simulink model "Proyecto_Final"  (R2025a)
settings: Solver=VariableStepAuto  StartTime=0.0  StopTime=10  RelTol=1e-3
undefined symbols (not defined in the file): X, Y, Z
libraries: fl_lib x336, nesl_utility x145, ee_lib x106, sm_lib x90, slpidlib x10
(part 2 of 13)

== system Proyecto_Final/Motor DC  ,Puente H y buck1 ==
  PS-Simulink Converter : nesl_utility/PS-Simulink Converter  PhysicalDomain=network_engine_domain  SubClassName=ps_output  LeftPortType=input  RightPortType=output  PseudoPeriodic=off  Frequencies=[]  VectorFormat=inherit  Unit=inherit  AffineConversion=off
  Scope3 : Scope
      settings: ActiveDisplayYMinimum=-1  ActiveDisplayYMaximum=1  DataLoggingVariableName=ScopeData11
  Subsystem : Subsystem
      settings: PortSchema="{\"entries\":[{\"content\":{\"sides\":[{\"content\":{\"connectorIds\":[\"LConn1\",\"LConn2\"]},\"type\":\"ConnectorPlacement.EquallySpacedRectSide\",\"uuid\":\"ba5a9f42-2585-4bfc-af33-0b26837d5344\"},{\"content\":{\"side\":\"RIGHT\"},\"type\":\"ConnectorPlacement.EquallySpacedRectSide\",\"uuid\":\"d3378d1a-9a35-4354-ae00-36e97aeae038\"},{\"content\":{\"connectorIds\":[\"LConn3\",\"LConn4\"],\"side\":\"TOP\"},\"type\":\"ConnectorPlacement.EquallySpacedRectSide\",\"uuid\":\"d7bba951-f995-49de-af79-0de620a32033\"}]},\"type\":\"ConnectorPlacement.EquallySpacedConnector\",\"uuid\":\"942587ed-ad52-4230-b73d-c158f6029d96\"}],\"packageUris\":[\"http://schema.mathworks.com/mf0/Connector/R2020b\"],\"version\":\"1.0\"}"
      mask Display: image('motordc.png');
  Subsystem1 : Subsystem
      mask Display: image('puenteh.png');
  Subsystem2 : Subsystem
      settings: PortSchema="{\"entries\":[{\"content\":{\"sides\":[{\"content\":{},\"type\":\"ConnectorPlacement.EquallySpacedRectSide\",\"uuid\":\"c0475787-e2dd-413a-bffe-1d488c503390\"},{\"content\":{\"connectorIds\":[\"RConn1\",\"RConn2\"],\"side\":\"RIGHT\"},\"type\":\"ConnectorPlacement.EquallySpacedRectSide\",\"uuid\":\"7136259c-9599-4eb8-8e1f-6288fad3fd4d\"},{\"content\":{\"side\":\"TOP\"},\"type\":\"ConnectorPlacement.EquallySpacedRectSide\",\"uuid\":\"c12a757b-7dec-4835-b4c8-0dd09d9bf8df\"},{\"content\":{\"connectorIds\":[\"RConn3\"],\"side\":\"BOTTOM\"},\"type\":\"ConnectorPlacement.EquallySpacedRectSide\",\"uuid\":\"8c834916-1092-4edf-bbd6-cfa333fcf008\"}]},\"type\":\"ConnectorPlacement.EquallySpacedConnector\",\"uuid\":\"4818e542-4a83-49f7-b80e-d9385aa09b38\"}],\"packageUris\":[\"http://schema.mathworks.com/mf0/Connector/R2020b\"],\"version\":\"1.0\"}"
      mask Display: image('buck.jpg');
  Voltage Sensor1 : fl_lib/Electrical/Electrical Sensors/Voltage Sensor
  w : PMIOPort  Side=Right
  t : PMIOPort  Port=2  Side=Right
  Lazo : PMIOPort  Port=3  Side=Right
  wires:
  PS-Simulink Converter/1 -> Scope3/1
  connections:
  Subsystem1/LConn1 -- Voltage Sensor1/LConn1 -- Subsystem2/RConn1
  Voltage Sensor1/RConn2 -- Subsystem1/LConn2 -- Subsystem2/RConn2
  Voltage Sensor1/RConn1 -- PS-Simulink Converter/LConn1
  w/RConn1 -- Subsystem/LConn4
  Subsystem/LConn3 -- t/RConn1
  Subsystem1/RConn1 -- Subsystem/LConn1
  Subsystem1/RConn2 -- Subsystem/LConn2
  Lazo/RConn1 -- Subsystem2/RConn3

== system Proyecto_Final/Motor DC  ,Puente H y buck2 ==
  PS-Simulink Converter : nesl_utility/PS-Simulink Converter  PhysicalDomain=network_engine_domain  SubClassName=ps_output  LeftPortType=input  RightPortType=output  PseudoPeriodic=off  Frequencies=[]  VectorFormat=inherit  Unit=inherit  AffineConversion=off
  Scope3 : Scope
      settings: ActiveDisplayYMinimum=-166.62843332082716  ActiveDisplayYMaximum=1034.7868051822825  DataLoggingVariableName=ScopeData33
  Subsystem : Subsystem
      settings: PortSchema="{\"entries\":[{\"content\":{\"sides\":[{\"content\":{\"connectorIds\":[\"LConn1\",\"LConn2\"]},\"type\":\"ConnectorPlacement.EquallySpacedRectSide\",\"uuid\":\"ba5a9f42-2585-4bfc-af33-0b26837d5344\"},{\"content\":{\"side\":\"RIGHT\"},\"type\":\"ConnectorPlacement.EquallySpacedRectSide\",\"uuid\":\"d3378d1a-9a35-4354-ae00-36e97aeae038\"},{\"content\":{\"connectorIds\":[\"LConn3\",\"LConn4\"],\"side\":\"TOP\"},\"type\":\"ConnectorPlacement.EquallySpacedRectSide\",\"uuid\":\"d7bba951-f995-49de-af79-0de620a32033\"}]},\"type\":\"ConnectorPlacement.EquallySpacedConnector\",\"uuid\":\"942587ed-ad52-4230-b73d-c158f6029d96\"}],\"packageUris\":[\"http://schema.mathworks.com/mf0/Connector/R2020b\"],\"version\":\"1.0\"}"
      mask Display: image('motordc.png');
  Subsystem1 : Subsystem
      mask Display: image('puenteh.png');
  Subsystem2 : Subsystem
      settings: PortSchema="{\"entries\":[{\"content\":{\"sides\":[{\"content\":{},\"type\":\"ConnectorPlacement.EquallySpacedRectSide\",\"uuid\":\"c0475787-e2dd-413a-bffe-1d488c503390\"},{\"content\":{\"connectorIds\":[\"RConn1\",\"RConn2\"],\"side\":\"RIGHT\"},\"type\":\"ConnectorPlacement.EquallySpacedRectSide\",\"uuid\":\"7136259c-9599-4eb8-8e1f-6288fad3fd4d\"},{\"content\":{\"side\":\"TOP\"},\"type\":\"ConnectorPlacement.EquallySpacedRectSide\",\"uuid\":\"c12a757b-7dec-4835-b4c8-0dd09d9bf8df\"},{\"content\":{\"connectorIds\":[\"RConn3\"],\"side\":\"BOTTOM\"},\"type\":\"ConnectorPlacement.EquallySpacedRectSide\",\"uuid\":\"8c834916-1092-4edf-bbd6-cfa333fcf008\"}]},\"type\":\"ConnectorPlacement.EquallySpacedConnector\",\"uuid\":\"4818e542-4a83-49f7-b80e-d9385aa09b38\"}],\"packageUris\":[\"http://schema.mathworks.com/mf0/Connector/R2020b\"],\"version\":\"1.0\"}"
      mask Display: image('buck.jpg');
  Voltage Sensor1 : fl_lib/Electrical/Electrical Sensors/Voltage Sensor
  w : PMIOPort  Side=Right
  t : PMIOPort  Port=2  Side=Right
  Lazo : PMIOPort  Port=3  Side=Right
  wires:
  PS-Simulink Converter/1 -> Scope3/1
  connections:
  Subsystem1/LConn2 -- Subsystem2/RConn2 -- Voltage Sensor1/RConn2
  Subsystem1/LConn1 -- Voltage Sensor1/LConn1 -- Subsystem2/RConn1
  Lazo/RConn1 -- Subsystem2/RConn3
  Subsystem1/RConn2 -- Subsystem/LConn2
  Subsystem/LConn3 -- t/RConn1
  Voltage Sensor1/RConn1 -- PS-Simulink Converter/LConn1
  w/RConn1 -- Subsystem/LConn4
  Subsystem1/RConn1 -- Subsystem/LConn1

== system Proyecto_Final/Motor DC  ,Puente H y buck3 ==
  PS-Simulink Converter : nesl_utility/PS-Simulink Converter  PhysicalDomain=network_engine_domain  SubClassName=ps_output  LeftPortType=input  RightPortType=output  PseudoPeriodic=off  Frequencies=[]  VectorFormat=inherit  Unit=inherit  AffineConversion=off
  Scope3 : Scope
      settings: ActiveDisplayYMinimum=-1  ActiveDisplayYMaximum=1  DataLoggingVariableName=ScopeData11
  Subsystem : Subsystem
      settings: PortSchema="{\"entries\":[{\"content\":{\"sides\":[{\"content\":{\"connectorIds\":[\"LConn1\",\"LConn2\"]},\"type\":\"ConnectorPlacement.EquallySpacedRectSide\",\"uuid\":\"ba5a9f42-2585-4bfc-af33-0b26837d5344\"},{\"content\":{\"side\":\"RIGHT\"},\"type\":\"ConnectorPlacement.EquallySpacedRectSide\",\"uuid\":\"d3378d1a-9a35-4354-ae00-36e97aeae038\"},{\"content\":{\"connectorIds\":[\"LConn3\",\"LConn4\"],\"side\":\"TOP\"},\"type\":\"ConnectorPlacement.EquallySpacedRectSide\",\"uuid\":\"d7bba951-f995-49de-af79-0de620a32033\"}]},\"type\":\"ConnectorPlacement.EquallySpacedConnector\",\"uuid\":\"942587ed-ad52-4230-b73d-c158f6029d96\"}],\"packageUris\":[\"http://schema.mathworks.com/mf0/Connector/R2020b\"],\"version\":\"1.0\"}"
      mask Display: image('motordc.png');
  Subsystem1 : Subsystem
      mask Display: image('puenteh.png');
  Subsystem2 : Subsystem
      settings: PortSchema="{\"entries\":[{\"content\":{\"sides\":[{\"content\":{},\"type\":\"ConnectorPlacement.EquallySpacedRectSide\",\"uuid\":\"c0475787-e2dd-413a-bffe-1d488c503390\"},{\"content\":{\"connectorIds\":[\"RConn1\",\"RConn2\"],\"side\":\"RIGHT\"},\"type\":\"ConnectorPlacement.EquallySpacedRectSide\",\"uuid\":\"7136259c-9599-4eb8-8e1f-6288fad3fd4d\"},{\"content\":{\"side\":\"TOP\"},\"type\":\"ConnectorPlacement.EquallySpacedRectSide\",\"uuid\":\"c12a757b-7dec-4835-b4c8-0dd09d9bf8df\"},{\"content\":{\"connectorIds\":[\"RConn3\"],\"side\":\"BOTTOM\"},\"type\":\"ConnectorPlacement.EquallySpacedRectSide\",\"uuid\":\"8c834916-1092-4edf-bbd6-cfa333fcf008\"}]},\"type\":\"ConnectorPlacement.EquallySpacedConnector\",\"uuid\":\"4818e542-4a83-49f7-b80e-d9385aa09b38\"}],\"packageUris\":[\"http://schema.mathworks.com/mf0/Connector/R2020b\"],\"version\":\"1.0\"}"
      mask Display: image('buck.jpg');
  Voltage Sensor1 : fl_lib/Electrical/Electrical Sensors/Voltage Sensor
  w : PMIOPort  Side=Right
  t : PMIOPort  Port=2  Side=Right
  Lazo : PMIOPort  Port=3  Side=Right
  wires:
  PS-Simulink Converter/1 -> Scope3/1
  connections:
  Voltage Sensor1/LConn1 -- Subsystem2/RConn1 -- Subsystem1/LConn1
  Voltage Sensor1/RConn2 -- Subsystem1/LConn2 -- Subsystem2/RConn2
  Voltage Sensor1/RConn1 -- PS-Simulink Converter/LConn1
  w/RConn1 -- Subsystem/LConn4
  Subsystem/LConn3 -- t/RConn1
  Subsystem1/RConn1 -- Subsystem/LConn1
  Subsystem1/RConn2 -- Subsystem/LConn2
  Lazo/RConn1 -- Subsystem2/RConn3

== system Proyecto_Final/Motor DC  ,Puente H y buck4 ==
  PS-Simulink Converter : nesl_utility/PS-Simulink Converter  PhysicalDomain=network_engine_domain  SubClassName=ps_output  LeftPortType=input  RightPortType=output  PseudoPeriodic=off  Frequencies=[]  VectorFormat=inherit  Unit=inherit  AffineConversion=off
  Scope3 : Scope
      settings: ActiveDisplayYMinimum=-166.62843332082716  ActiveDisplayYMaximum=1034.7868051822825  DataLoggingVariableName=ScopeData33
  Subsystem : Subsystem
      settings: PortSchema="{\"entries\":[{\"content\":{\"sides\":[{\"content\":{\"connectorIds\":[\"LConn1\",\"LConn2\"]},\"type\":\"ConnectorPlacement.EquallySpacedRectSide\",\"uuid\":\"ba5a9f42-2585-4bfc-af33-0b26837d5344\"},{\"content\":{\"side\":\"RIGHT\"},\"type\":\"ConnectorPlacement.EquallySpacedRectSide\",\"uuid\":\"d3378d1a-9a35-4354-ae00-36e97aeae038\"},{\"content\":{\"connectorIds\":[\"LConn3\",\"LConn4\"],\"side\":\"TOP\"},\"type\":\"ConnectorPlacement.EquallySpacedRectSide\",\"uuid\":\"d7bba951-f995-49de-af79-0de620a32033\"}]},\"type\":\"ConnectorPlacement.EquallySpacedConnector\",\"uuid\":\"942587ed-ad52-4230-b73d-c158f6029d96\"}],\"packageUris\":[\"http://schema.mathworks.com/mf0/Connector/R2020b\"],\"version\":\"1.0\"}"
      mask Display: image('motordc.png');
  Subsystem1 : Subsystem
      mask Display: image('puenteh.png');
  Subsystem2 : Subsystem
      settings: PortSchema="{\"entries\":[{\"content\":{\"sides\":[{\"content\":{},\"type\":\"ConnectorPlacement.EquallySpacedRectSide\",\"uuid\":\"c0475787-e2dd-413a-bffe-1d488c503390\"},{\"content\":{\"connectorIds\":[\"RConn1\",\"RConn2\"],\"side\":\"RIGHT\"},\"type\":\"ConnectorPlacement.EquallySpacedRectSide\",\"uuid\":\"7136259c-9599-4eb8-8e1f-6288fad3fd4d\"},{\"content\":{\"side\":\"TOP\"},\"type\":\"ConnectorPlacement.EquallySpacedRectSide\",\"uuid\":\"c12a757b-7dec-4835-b4c8-0dd09d9bf8df\"},{\"content\":{\"connectorIds\":[\"RConn3\"],\"side\":\"BOTTOM\"},\"type\":\"ConnectorPlacement.EquallySpacedRectSide\",\"uuid\":\"8c834916-1092-4edf-bbd6-cfa333fcf008\"}]},\"type\":\"ConnectorPlacement.EquallySpacedConnector\",\"uuid\":\"4818e542-4a83-49f7-b80e-d9385aa09b38\"}],\"packageUris\":[\"http://schema.mathworks.com/mf0/Connector/R2020b\"],\"version\":\"1.0\"}"
      mask Display: image('buck.jpg');
  Voltage Sensor1 : fl_lib/Electrical/Electrical Sensors/Voltage Sensor
  w : PMIOPort  Side=Right
  t : PMIOPort  Port=2  Side=Right
  Lazo : PMIOPort  Port=3  Side=Right
  wires:
  PS-Simulink Converter/1 -> Scope3/1
  connections:
  Subsystem2/RConn2 -- Voltage Sensor1/RConn2 -- Subsystem1/LConn2
  Voltage Sensor1/LConn1 -- Subsystem2/RConn1 -- Subsystem1/LConn1
  Lazo/RConn1 -- Subsystem2/RConn3
  Subsystem1/RConn2 -- Subsystem/LConn2
  Subsystem/LConn3 -- t/RConn1
  Voltage Sensor1/RConn1 -- PS-Simulink Converter/LConn1
  w/RConn1 -- Subsystem/LConn4
  Subsystem1/RConn1 -- Subsystem/LConn1

== system Proyecto_Final/Motor DC  ,Puente H y buck5 ==
  PS-Simulink Converter : nesl_utility/PS-Simulink Converter  PhysicalDomain=network_engine_domain  SubClassName=ps_output  LeftPortType=input  RightPortType=output  PseudoPeriodic=off  Frequencies=[]  VectorFormat=inherit  Unit=inherit  AffineConversion=off
  Scope3 : Scope
      settings: ActiveDisplayYMinimum=-166.62843332082716  ActiveDisplayYMaximum=1034.7868051822825  DataLoggingVariableName=ScopeData34
  Subsystem : Subsystem
      settings: PortSchema="{\"entries\":[{\"content\":{\"sides\":[{\"content\":{\"connectorIds\":[\"LConn1\",\"LConn2\"]},\"type\":\"ConnectorPlacement.EquallySpacedRectSide\",\"uuid\":\"ba5a9f42-2585-4bfc-af33-0b26837d5344\"},{\"content\":{\"side\":\"RIGHT\"},\"type\":\"ConnectorPlacement.EquallySpacedRectSide\",\"uuid\":\"d3378d1a-9a35-4354-ae00-36e97aeae038\"},{\"content\":{\"connectorIds\":[\"LConn3\",\"LConn4\"],\"side\":\"TOP\"},\"type\":\"ConnectorPlacement.EquallySpacedRectSide\",\"uuid\":\"d7bba951-f995-49de-af79-0de620a32033\"}]},\"type\":\"ConnectorPlacement.EquallySpacedConnector\",\"uuid\":\"942587ed-ad52-4230-b73d-c158f6029d96\"}],\"packageUris\":[\"http://schema.mathworks.com/mf0/Connector/R2020b\"],\"version\":\"1.0\"}"
      mask Display: image('motordc.png');
  Subsystem1 : Subsystem
      mask Display: image('puenteh.png');
  Subsystem2 : Subsystem
      settings: PortSchema="{\"entries\":[{\"content\":{\"sides\":[{\"content\":{},\"type\":\"ConnectorPlacement.EquallySpacedRectSide\",\"uuid\":\"c0475787-e2dd-413a-bffe-1d488c503390\"},{\"content\":{\"connectorIds\":[\"RConn1\",\"RConn2\"],\"side\":\"RIGHT\"},\"type\":\"ConnectorPlacement.EquallySpacedRectSide\",\"uuid\":\"7136259c-9599-4eb8-8e1f-6288fad3fd4d\"},{\"content\":{\"side\":\"TOP\"},\"type\":\"ConnectorPlacement.EquallySpacedRectSide\",\"uuid\":\"c12a757b-7dec-4835-b4c8-0dd09d9bf8df\"},{\"content\":{\"connectorIds\":[\"RConn3\"],\"side\":\"BOTTOM\"},\"type\":\"ConnectorPlacement.EquallySpacedRectSide\",\"uuid\":\"8c834916-1092-4edf-bbd6-cfa333fcf008\"}]},\"type\":\"ConnectorPlacement.EquallySpacedConnector\",\"uuid\":\"4818e542-4a83-49f7-b80e-d9385aa09b38\"}],\"packageUris\":[\"http://schema.mathworks.com/mf0/Connector/R2020b\"],\"version\":\"1.0\"}"
      mask Display: image('buck.jpg');
  Voltage Sensor1 : fl_lib/Electrical/Electrical Sensors/Voltage Sensor
  w : PMIOPort  Side=Right
  t : PMIOPort  Port=2  Side=Right
  Lazo : PMIOPort  Port=3  Side=Right
  wires:
  PS-Simulink Converter/1 -> Scope3/1
  connections:
  Subsystem2/RConn2 -- Voltage Sensor1/RConn2 -- Subsystem1/LConn2
  Voltage Sensor1/LConn1 -- Subsystem2/RConn1 -- Subsystem1/LConn1
  Lazo/RConn1 -- Subsystem2/RConn3
  Subsystem1/RConn2 -- Subsystem/LConn2
  Subsystem/LConn3 -- t/RConn1
  Voltage Sensor1/RConn1 -- PS-Simulink Converter/LConn1
  w/RConn1 -- Subsystem/LConn4
  Subsystem1/RConn1 -- Subsystem/LConn1

== system Proyecto_Final/Motor DC  ,Puente H y buck6 ==
  PS-Simulink Converter : nesl_utility/PS-Simulink Converter  PhysicalDomain=network_engine_domain  SubClassName=ps_output  LeftPortType=input  RightPortType=output  PseudoPeriodic=off  Frequencies=[]  VectorFormat=inherit  Unit=inherit  AffineConversion=off
  Scope3 : Scope
      settings: ActiveDisplayYMinimum=-166.62843332082716  ActiveDisplayYMaximum=1034.7868051822825  DataLoggingVariableName=ScopeData34
  Subsystem : Subsystem
      settings: PortSchema="{\"entries\":[{\"content\":{\"sides\":[{\"content\":{\"connectorIds\":[\"LConn1\",\"LConn2\"]},\"type\":\"ConnectorPlacement.EquallySpacedRectSide\",\"uuid\":\"ba5a9f42-2585-4bfc-af33-0b26837d5344\"},{\"content\":{\"side\":\"RIGHT\"},\"type\":\"ConnectorPlacement.EquallySpacedRectSide\",\"uuid\":\"d3378d1a-9a35-4354-ae00-36e97aeae038\"},{\"content\":{\"connectorIds\":[\"LConn3\",\"LConn4\"],\"side\":\"TOP\"},\"type\":\"ConnectorPlacement.EquallySpacedRectSide\",\"uuid\":\"d7bba951-f995-49de-af79-0de620a32033\"}]},\"type\":\"ConnectorPlacement.EquallySpacedConnector\",\"uuid\":\"942587ed-ad52-4230-b73d-c158f6029d96\"}],\"packageUris\":[\"http://schema.mathworks.com/mf0/Connector/R2020b\"],\"version\":\"1.0\"}"
      mask Display: image('motordc.png');
  Subsystem1 : Subsystem
      mask Display: image('puenteh.png');
  Subsystem2 : Subsystem
      settings: PortSchema="{\"entries\":[{\"content\":{\"sides\":[{\"content\":{},\"type\":\"ConnectorPlacement.EquallySpacedRectSide\",\"uuid\":\"c0475787-e2dd-413a-bffe-1d488c503390\"},{\"content\":{\"connectorIds\":[\"RConn1\",\"RConn2\"],\"side\":\"RIGHT\"},\"type\":\"ConnectorPlacement.EquallySpacedRectSide\",\"uuid\":\"7136259c-9599-4eb8-8e1f-6288fad3fd4d\"},{\"content\":{\"side\":\"TOP\"},\"type\":\"ConnectorPlacement.EquallySpacedRectSide\",\"uuid\":\"c12a757b-7dec-4835-b4c8-0dd09d9bf8df\"},{\"content\":{\"connectorIds\":[\"RConn3\"],\"side\":\"BOTTOM\"},\"type\":\"ConnectorPlacement.EquallySpacedRectSide\",\"uuid\":\"8c834916-1092-4edf-bbd6-cfa333fcf008\"}]},\"type\":\"ConnectorPlacement.EquallySpacedConnector\",\"uuid\":\"4818e542-4a83-49f7-b80e-d9385aa09b38\"}],\"packageUris\":[\"http://schema.mathworks.com/mf0/Connector/R2020b\"],\"version\":\"1.0\"}"
      mask Display: image('buck.jpg');
  Voltage Sensor1 : fl_lib/Electrical/Electrical Sensors/Voltage Sensor
  w : PMIOPort  Side=Right
  t : PMIOPort  Port=2  Side=Right
  Lazo : PMIOPort  Port=3  Side=Right
  wires:
  PS-Simulink Converter/1 -> Scope3/1
  connections:
  Subsystem1/LConn2 -- Subsystem2/RConn2 -- Voltage Sensor1/RConn2
  Subsystem1/LConn1 -- Voltage Sensor1/LConn1 -- Subsystem2/RConn1
  Lazo/RConn1 -- Subsystem2/RConn3
  Subsystem1/RConn2 -- Subsystem/LConn2
  Subsystem/LConn3 -- t/RConn1
  Voltage Sensor1/RConn1 -- PS-Simulink Converter/LConn1
  w/RConn1 -- Subsystem/LConn4
  Subsystem1/RConn1 -- Subsystem/LConn1

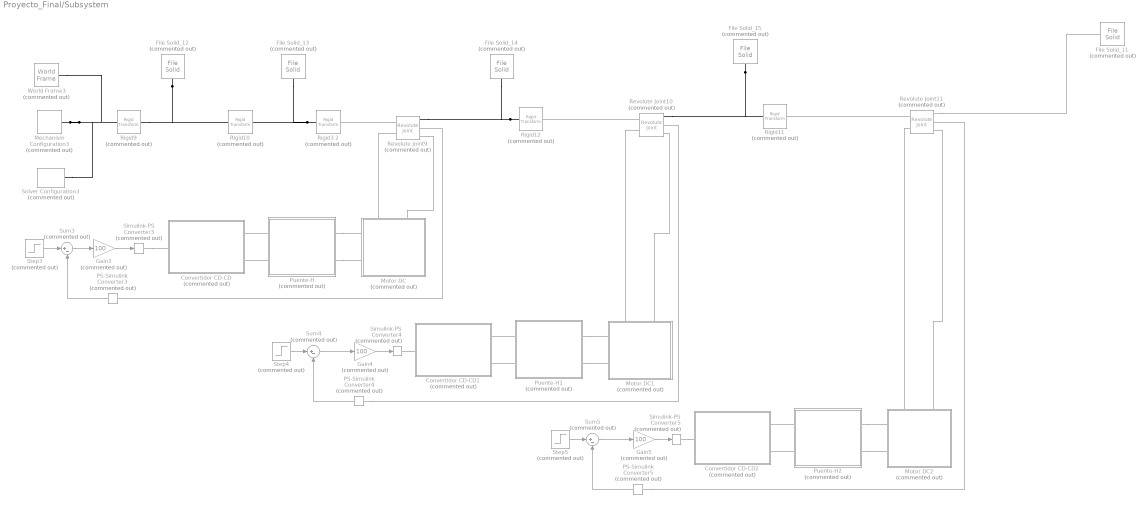
== system Proyecto_Final/Subsystem ==
  Convertidor CD-CD : Subsystem  Commented=on
      mask Display: image('buck.jpg');
  Convertidor CD-CD1 : Subsystem  Commented=on
      mask Display: image('buck.jpg');
  Convertidor CD-CD2 : Subsystem  Commented=on
      mask Display: image('buck.jpg');
  File Solid_11 : sm_lib/Body Elements/File Solid  Commented=on  ExtGeomFileName=C:\Users\jlope\Downloads\CUCEI TAREAS\Semi modelado\Proyecto Final\PIEZAS BUENAS\P5.STEP  UnitType=FromFile  ExtGeomFileUnits=m  StepReaderType=HEX  ExportConvexHullGeometry=off  InertiaType=CalculateFromGeometry  BasedOnType=Mass  Density=1000  DensityUnits=kg/m^3  Mass=1  MassUnits=kg  CenterOfMass=[0 0 0]  CenterOfMassUnits=m  MomentsOfInertia=[1 1 1]  MomentsOfInertiaUnits=kg*m^2  ProductsOfInertia=[0 0 0]  ProductsOfInertiaUnits=kg*m^2  GraphicType=FromGeometry  MarkerShape=Sphere  MarkerSize=10  GraphicVisPropType=SimpleVisualProperties  GraphicDiffuseColor=[0.5 0.5 0.5]  GraphicOpacity=1  GraphicSpecularColor=[0.5 0.5 0.5 1.0]  GraphicAmbientColor=[0.15 0.15 0.15 1.0]  GraphicEmissiveColor=[0.0 0.0 0.0 1.0]  GraphicShininess=75  DoExposeReferenceFrame=on  SerializedFrames=<Frames/>
  File Solid_12 : sm_lib/Body Elements/File Solid  Commented=on  ExtGeomFileName=C:\Users\jlope\Downloads\CUCEI TAREAS\Semi modelado\Proyecto Final\PIEZAS BUENAS\P1.STEP  UnitType=Custom  ExtGeomFileUnits=mm  StepReaderType=HEX  ExportConvexHullGeometry=off  InertiaType=CalculateFromGeometry  BasedOnType=Mass  Density=1000  DensityUnits=kg/m^3  Mass=1  MassUnits=kg  CenterOfMass=[0 0 0]  CenterOfMassUnits=m  MomentsOfInertia=[1 1 1]  MomentsOfInertiaUnits=kg*m^2  ProductsOfInertia=[0 0 0]  ProductsOfInertiaUnits=kg*m^2  GraphicType=FromGeometry  MarkerShape=Sphere  MarkerSize=10  GraphicVisPropType=SimpleVisualProperties  GraphicDiffuseColor=[0.2784 0.298 0.3059]  GraphicOpacity=1  GraphicSpecularColor=[0.5 0.5 0.5 1.0]  GraphicAmbientColor=[0.15 0.15 0.15 1.0]  GraphicEmissiveColor=[0.0 0.0 0.0 1.0]  GraphicShininess=75  DoExposeReferenceFrame=on  SerializedFrames=<Frames/>
  File Solid_13 : sm_lib/Body Elements/File Solid  Commented=on  ExtGeomFileName=C:\Users\jlope\Downloads\CUCEI TAREAS\Semi modelado\Proyecto Final\PIEZAS BUENAS\P2.STEP  UnitType=FromFile  ExtGeomFileUnits=m  StepReaderType=HEX  ExportConvexHullGeometry=off  InertiaType=CalculateFromGeometry  BasedOnType=Mass  Density=1000  DensityUnits=kg/m^3  Mass=1  MassUnits=kg  CenterOfMass=[0 0 0]  CenterOfMassUnits=m  MomentsOfInertia=[1 1 1]  MomentsOfInertiaUnits=kg*m^2  ProductsOfInertia=[0 0 0]  ProductsOfInertiaUnits=kg*m^2  GraphicType=FromGeometry  MarkerShape=Sphere  MarkerSize=10  GraphicVisPropType=SimpleVisualProperties  GraphicDiffuseColor=[0.5 0.5 0.5]  GraphicOpacity=1  GraphicSpecularColor=[0.5 0.5 0.5 1.0]  GraphicAmbientColor=[0.15 0.15 0.15 1.0]  GraphicEmissiveColor=[0.0 0.0 0.0 1.0]  GraphicShininess=75  DoExposeReferenceFrame=on  SerializedFrames=<Frames/>
  File Solid_14 : sm_lib/Body Elements/File Solid  Commented=on  ExtGeomFileName=C:\Users\jlope\Downloads\CUCEI TAREAS\Semi modelado\Proyecto Final\PIEZAS BUENAS\P3.STEP  UnitType=FromFile  ExtGeomFileUnits=m  StepReaderType=HEX  ExportConvexHullGeometry=off  InertiaType=CalculateFromGeometry  BasedOnType=Mass  Density=1000  DensityUnits=kg/m^3  Mass=1  MassUnits=kg  CenterOfMass=[0 0 0]  CenterOfMassUnits=m  MomentsOfInertia=[1 1 1]  MomentsOfInertiaUnits=kg*m^2  ProductsOfInertia=[0 0 0]  ProductsOfInertiaUnits=kg*m^2  GraphicType=FromGeometry  MarkerShape=Sphere  MarkerSize=10  GraphicVisPropType=SimpleVisualProperties  GraphicDiffuseColor=[0.5 0.5 0.5]  GraphicOpacity=1  GraphicSpecularColor=[0.5 0.5 0.5 1.0]  GraphicAmbientColor=[0.15 0.15 0.15 1.0]  GraphicEmissiveColor=[0.0 0.0 0.0 1.0]  GraphicShininess=75  DoExposeReferenceFrame=on  SerializedFrames=<Frames/>
  File Solid_15 : sm_lib/Body Elements/File Solid  Commented=on  ExtGeomFileName=C:\Users\jlope\Downloads\CUCEI TAREAS\Semi modelado\Proyecto Final\PIEZAS BUENAS\P4.STEP  UnitType=FromFile  ExtGeomFileUnits=m  StepReaderType=HEX  ExportConvexHullGeometry=off  InertiaType=CalculateFromGeometry  BasedOnType=Mass  Density=1000  DensityUnits=kg/m^3  Mass=1  MassUnits=kg  CenterOfMass=[0 0 0]  CenterOfMassUnits=m  MomentsOfInertia=[1 1 1]  MomentsOfInertiaUnits=kg*m^2  ProductsOfInertia=[0 0 0]  ProductsOfInertiaUnits=kg*m^2  GraphicType=FromGeometry  MarkerShape=Sphere  MarkerSize=10  GraphicVisPropType=SimpleVisualProperties  GraphicDiffuseColor=[0.5 0.5 0.5]  GraphicOpacity=1  GraphicSpecularColor=[0.5 0.5 0.5 1.0]  GraphicAmbientColor=[0.15 0.15 0.15 1.0]  GraphicEmissiveColor=[0.0 0.0 0.0 1.0]  GraphicShininess=75  DoExposeReferenceFrame=on  SerializedFrames=<Frames/>
  Gain3 : Gain  Commented=on  Gain=100
  Gain4 : Gain  Commented=on  Gain=100
  Gain5 : Gain  Commented=on  Gain=100
  Mechanism Configuration3 : sm_lib/Utilities/Mechanism Configuration  Commented=on  UniformGravity=Constant  GravityVector=[0 0 -9.80665]  GravityVectorUnits=m/s^2  LinearizationDelta=0.001  JointModeTransitionNonlinearIterations=2
  Motor DC : Subsystem  Commented=on
      settings: PortSchema="{\"entries\":[{\"content\":{\"sides\":[{\"content\":{\"connectorIds\":[\"LConn1\",\"LConn2\"]},\"type\":\"ConnectorPlacement.EquallySpacedRectSide\",\"uuid\":\"c5bd0a00-8d67-4fda-b008-e2a82d6ca81a\"},{\"content\":{\"side\":\"RIGHT\"},\"type\":\"ConnectorPlacement.EquallySpacedRectSide\",\"uuid\":\"40c2c73a-7123-476f-ac1e-8adf2ef682b4\"},{\"content\":{\"connectorIds\":[\"LConn3\",\"LConn4\"],\"side\":\"TOP\"},\"type\":\"ConnectorPlacement.EquallySpacedRectSide\",\"uuid\":\"cff9c687-df8a-4f8c-81b3-13e4060bdf9d\"}]},\"type\":\"ConnectorPlacement.EquallySpacedConnector\",\"uuid\":\"a20321ca-7a3c-4909-bd97-df50c3917fb4\"}],\"packageUris\":[\"http://schema.mathworks.com/mf0/Connector/R2020b\"],\"version\":\"1.0\"}"
      mask Display: image('motordc.png');
  Motor DC1 : Subsystem  Commented=on
      settings: PortSchema="{\"entries\":[{\"content\":{\"sides\":[{\"content\":{\"connectorIds\":[\"LConn1\",\"LConn2\"]},\"type\":\"ConnectorPlacement.EquallySpacedRectSide\",\"uuid\":\"c5bd0a00-8d67-4fda-b008-e2a82d6ca81a\"},{\"content\":{\"side\":\"RIGHT\"},\"type\":\"ConnectorPlacement.EquallySpacedRectSide\",\"uuid\":\"40c2c73a-7123-476f-ac1e-8adf2ef682b4\"},{\"content\":{\"connectorIds\":[\"LConn3\",\"LConn4\"],\"side\":\"TOP\"},\"type\":\"ConnectorPlacement.EquallySpacedRectSide\",\"uuid\":\"cff9c687-df8a-4f8c-81b3-13e4060bdf9d\"}]},\"type\":\"ConnectorPlacement.EquallySpacedConnector\",\"uuid\":\"a20321ca-7a3c-4909-bd97-df50c3917fb4\"}],\"packageUris\":[\"http://schema.mathworks.com/mf0/Connector/R2020b\"],\"version\":\"1.0\"}"
      mask Display: image('motordc.png');
  Motor DC2 : Subsystem  Commented=on
      settings: PortSchema="{\"entries\":[{\"content\":{\"sides\":[{\"content\":{\"connectorIds\":[\"LConn1\",\"LConn2\"]},\"type\":\"ConnectorPlacement.EquallySpacedRectSide\",\"uuid\":\"c5bd0a00-8d67-4fda-b008-e2a82d6ca81a\"},{\"content\":{\"side\":\"RIGHT\"},\"type\":\"ConnectorPlacement.EquallySpacedRectSide\",\"uuid\":\"40c2c73a-7123-476f-ac1e-8adf2ef682b4\"},{\"content\":{\"connectorIds\":[\"LConn3\",\"LConn4\"],\"side\":\"TOP\"},\"type\":\"ConnectorPlacement.EquallySpacedRectSide\",\"uuid\":\"cff9c687-df8a-4f8c-81b3-13e4060bdf9d\"}]},\"type\":\"ConnectorPlacement.EquallySpacedConnector\",\"uuid\":\"a20321ca-7a3c-4909-bd97-df50c3917fb4\"}],\"packageUris\":[\"http://schema.mathworks.com/mf0/Connector/R2020b\"],\"version\":\"1.0\"}"
      mask Display: image('motordc.png');
  PS-Simulink Converter3 : nesl_utility/PS-Simulink Converter  Commented=on  PhysicalDomain=network_engine_domain  SubClassName=ps_output  LeftPortType=input  RightPortType=output  PseudoPeriodic=off  Frequencies=[]  VectorFormat=inherit  Unit=inherit  AffineConversion=off
  PS-Simulink Converter4 : nesl_utility/PS-Simulink Converter  Commented=on  PhysicalDomain=network_engine_domain  SubClassName=ps_output  LeftPortType=input  RightPortType=output  PseudoPeriodic=off  Frequencies=[]  VectorFormat=inherit  Unit=inherit  AffineConversion=off
  PS-Simulink Converter5 : nesl_utility/PS-Simulink Converter  Commented=on  PhysicalDomain=network_engine_domain  SubClassName=ps_output  LeftPortType=input  RightPortType=output  PseudoPeriodic=off  Frequencies=[]  VectorFormat=inherit  Unit=inherit  AffineConversion=off
  Puente-H : Subsystem  Commented=on
      mask Display: image('puenteh.png');
  Puente-H1 : Subsystem  Commented=on
      mask Display: image('puenteh.png');
  Puente-H2 : Subsystem  Commented=on
      mask Display: image('puenteh.png');
  Revolute Joint10 : sm_lib/Joints/Revolute Joint  Commented=on  JointMode=Normal  CompositeWrenchDir=FollowerOnBase  CompositeWrenchFrame=BaseFrame  SenseConstraintForce=off  SenseConstraintTorque=off  SenseTotalForce=off  SenseTotalTorque=off  PositionTargetSpecify=off  PositionTargetPriority=High  PositionTargetValue=0  PositionTargetValueUnits=deg  VelocityTargetSpecify=off  VelocityTargetPriority=High  VelocityTargetValue=0  VelocityTargetValueUnits=deg/s  EquilibriumPosition=0  EquilibriumPositionUnits=deg  SpringStiffness=0  SpringStiffnessUnits=N*m/deg  DampingCoefficient=0  DampingCoefficientUnits=N*m/(deg/s)  LowerLimitSpecify=off  LowerLimitBound=-90  LowerLimitBoundUnits=deg  LowerLimitStiffness=1e4  LowerLimitStiffnessUnits=N*m/deg  LowerLimitDamping=10  LowerLimitDampingUnits=N*m/(deg/s)  LowerLimitTransitionRegionWidth=0.1  LowerLimitTransitionRegionWidthUnits=deg  UpperLimitSpecify=off  UpperLimitBound=90  UpperLimitBoundUnits=deg  UpperLimitStiffness=1e4  UpperLimitStiffnessUnits=N*m/deg  UpperLimitDamping=10  UpperLimitDampingUnits=N*m/(deg/s)  UpperLimitTransitionRegionWidth=0.1  UpperLimitTransitionRegionWidthUnits=deg  TorqueActuationMode=InputTorque  MotionActuationMode=ComputedMotion  SensePosition=on  SenseVelocity=on  SenseAcceleration=off  SenseTorqueForce=off  SenseLowerLimitTorqueForce=off  SenseUpperLimitTorqueForce=off
  Revolute Joint11 : sm_lib/Joints/Revolute Joint  Commented=on  JointMode=Normal  CompositeWrenchDir=FollowerOnBase  CompositeWrenchFrame=BaseFrame  SenseConstraintForce=off  SenseConstraintTorque=off  SenseTotalForce=off  SenseTotalTorque=off  PositionTargetSpecify=off  PositionTargetPriority=High  PositionTargetValue=0  PositionTargetValueUnits=deg  VelocityTargetSpecify=off  VelocityTargetPriority=High  VelocityTargetValue=0  VelocityTargetValueUnits=deg/s  EquilibriumPosition=0  EquilibriumPositionUnits=deg  SpringStiffness=0  SpringStiffnessUnits=N*m/deg  DampingCoefficient=0  DampingCoefficientUnits=N*m/(deg/s)  LowerLimitSpecify=off  LowerLimitBound=-90  LowerLimitBoundUnits=deg  LowerLimitStiffness=1e4  LowerLimitStiffnessUnits=N*m/deg  LowerLimitDamping=10  LowerLimitDampingUnits=N*m/(deg/s)  LowerLimitTransitionRegionWidth=0.1  LowerLimitTransitionRegionWidthUnits=deg  UpperLimitSpecify=off  UpperLimitBound=90  UpperLimitBoundUnits=deg  UpperLimitStiffness=1e4  UpperLimitStiffnessUnits=N*m/deg  UpperLimitDamping=10  UpperLimitDampingUnits=N*m/(deg/s)  UpperLimitTransitionRegionWidth=0.1  UpperLimitTransitionRegionWidthUnits=deg  TorqueActuationMode=InputTorque  MotionActuationMode=ComputedMotion  SensePosition=on  SenseVelocity=on  SenseAcceleration=off  SenseTorqueForce=off  SenseLowerLimitTorqueForce=off  SenseUpperLimitTorqueForce=off
  Revolute Joint9 : sm_lib/Joints/Revolute Joint  Commented=on  JointMode=Normal  CompositeWrenchDir=FollowerOnBase  CompositeWrenchFrame=BaseFrame  SenseConstraintForce=off  SenseConstraintTorque=off  SenseTotalForce=off  SenseTotalTorque=off  PositionTargetSpecify=off  PositionTargetPriority=High  PositionTargetValue=0  PositionTargetValueUnits=deg  VelocityTargetSpecify=off  VelocityTargetPriority=High  VelocityTargetValue=0  VelocityTargetValueUnits=deg/s  EquilibriumPosition=0  EquilibriumPositionUnits=deg  SpringStiffness=0  SpringStiffnessUnits=N*m/deg  DampingCoefficient=0  DampingCoefficientUnits=N*m/(deg/s)  LowerLimitSpecify=off  LowerLimitBound=-90  LowerLimitBoundUnits=deg  LowerLimitStiffness=1e4  LowerLimitStiffnessUnits=N*m/deg  LowerLimitDamping=10  LowerLimitDampingUnits=N*m/(deg/s)  LowerLimitTransitionRegionWidth=0.1  LowerLimitTransitionRegionWidthUnits=deg  UpperLimitSpecify=off  UpperLimitBound=90  UpperLimitBoundUnits=deg  UpperLimitStiffness=1e4  UpperLimitStiffnessUnits=N*m/deg  UpperLimitDamping=10  UpperLimitDampingUnits=N*m/(deg/s)  UpperLimitTransitionRegionWidth=0.1  UpperLimitTransitionRegionWidthUnits=deg  TorqueActuationMode=InputTorque  MotionActuationMode=ComputedMotion  SensePosition=on  SenseVelocity=on  SenseAcceleration=off  SenseTorqueForce=off  SenseLowerLimitTorqueForce=off  SenseUpperLimitTorqueForce=off
  Rigid10 : sm_lib/Frames and Transforms/Rigid Transform  Commented=on  RotationMethod=None  FollAlignAxisA=+X  BaseAlignAxisA=+Y  FollAlignAxisB=+Y  BaseAlignAxisB=+Z  RotationStandardAxis=+X  RotationAngle=90  RotationAngleUnits=deg  RotationArbitraryAxis=[0 0 1]  RotationSequenceAxes=FollowerAxes  RotationSequence=XYX  RotationSequenceAngles=[0 0 0]  RotationSequenceAnglesUnits=deg  RotationMatrix=[1 0 0;0 1 0;0 0 1]  Quaternion=[1 0 0 0]  TranslationMethod=Cartesian  TranslationCartesianOffset=[0 180 0]  TranslationCartesianOffsetUnits=mm  TranslationStandardAxis=+Z  TranslationStandardOffset=0  TranslationStandardOffsetUnits=m  TranslationROffset=0  TranslationROffsetUnits=m  TranslationThetaOffset=0  TranslationThetaOffsetUnits=deg  TranslationZOffset=0  TranslationZOffsetUnits=m
  Rigid11 : sm_lib/Frames and Transforms/Rigid Transform  Commented=on  RotationMethod=None  FollAlignAxisA=+X  BaseAlignAxisA=+Y  FollAlignAxisB=+Y  BaseAlignAxisB=+Z  RotationStandardAxis=-X  RotationAngle=90  RotationAngleUnits=deg  RotationArbitraryAxis=[0 0 1]  RotationSequenceAxes=FollowerAxes  RotationSequence=XYX  RotationSequenceAngles=[0 0 0]  RotationSequenceAnglesUnits=deg  RotationMatrix=[1 0 0;0 1 0;0 0 1]  Quaternion=[1 0 0 0]  TranslationMethod=Cartesian  TranslationCartesianOffset=[-425 150 0]  TranslationCartesianOffsetUnits=mm  TranslationStandardAxis=+Z  TranslationStandardOffset=0  TranslationStandardOffsetUnits=m  TranslationROffset=0  TranslationROffsetUnits=m  TranslationThetaOffset=0  TranslationThetaOffsetUnits=deg  TranslationZOffset=0  TranslationZOffsetUnits=m
  Rigid12 : sm_lib/Frames and Transforms/Rigid Transform  Commented=on  RotationMethod=None  FollAlignAxisA=+X  BaseAlignAxisA=+Y  FollAlignAxisB=+Y  BaseAlignAxisB=+Z  RotationStandardAxis=-X  RotationAngle=90  RotationAngleUnits=deg  RotationArbitraryAxis=[0 0 1]  RotationSequenceAxes=FollowerAxes  RotationSequence=XYX  RotationSequenceAngles=[0 0 0]  RotationSequenceAnglesUnits=deg  RotationMatrix=[1 0 0;0 1 0;0 0 1]  Quaternion=[1 0 0 0]  TranslationMethod=Cartesian  TranslationCartesianOffset=[0 500 0]  TranslationCartesianOffsetUnits=mm  TranslationStandardAxis=+Z  TranslationStandardOffset=0  TranslationStandardOffsetUnits=m  TranslationROffset=0  TranslationROffsetUnits=m  TranslationThetaOffset=0  TranslationThetaOffsetUnits=deg  TranslationZOffset=0  TranslationZOffsetUnits=m
  Rigid3 2 : sm_lib/Frames and Transforms/Rigid Transform  Commented=on  RotationMethod=None  FollAlignAxisA=+X  BaseAlignAxisA=+Y  FollAlignAxisB=+Y  BaseAlignAxisB=+Z  RotationStandardAxis=+X  RotationAngle=90  RotationAngleUnits=deg  RotationArbitraryAxis=[0 0 1]  RotationSequenceAxes=FollowerAxes  RotationSequence=XYX  RotationSequenceAngles=[0 0 0]  RotationSequenceAnglesUnits=deg  RotationMatrix=[1 0 0;0 1 0;0 0 1]  Quaternion=[1 0 0 0]  TranslationMethod=Cartesian  TranslationCartesianOffset=[0 336 0]  TranslationCartesianOffsetUnits=mm  TranslationStandardAxis=+Z  TranslationStandardOffset=0  TranslationStandardOffsetUnits=m  TranslationROffset=0  TranslationROffsetUnits=m  TranslationThetaOffset=0  TranslationThetaOffsetUnits=deg  TranslationZOffset=0  TranslationZOffsetUnits=m
  Rigid9 : sm_lib/Frames and Transforms/Rigid Transform  Commented=on  RotationMethod=StandardAxis  FollAlignAxisA=+X  BaseAlignAxisA=+X  FollAlignAxisB=+Y  BaseAlignAxisB=+Z  RotationStandardAxis=+X  RotationAngle=90  RotationAngleUnits=deg  RotationArbitraryAxis=[0 0 1]  RotationSequenceAxes=FollowerAxes  RotationSequence=XYX  RotationSequenceAngles=[0 0 0]  RotationSequenceAnglesUnits=deg  RotationMatrix=[1 0 0;0 1 0;0 0 1]  Quaternion=[1 0 0 0]  TranslationMethod=None  TranslationCartesianOffset=[0 0 0]  TranslationCartesianOffsetUnits=m  TranslationStandardAxis=+Z  TranslationStandardOffset=0  TranslationStandardOffsetUnits=m  TranslationROffset=0  TranslationROffsetUnits=m  TranslationThetaOffset=0  TranslationThetaOffsetUnits=deg  TranslationZOffset=0  TranslationZOffsetUnits=m
  Simulink-PS Converter3 : nesl_utility/Simulink-PS Converter  Commented=on  PhysicalDomain=network_engine_domain  SubClassName=ps_input  LeftPortType=input  RightPortType=output  PseudoPeriodic=off  Frequencies=[]  NoiseDistribution=none  NoiseParameters=[]  Unit=1  AffineConversion=off  FilteringAndDerivatives=filter  SimscapeFilterOrder=1  InputFilterTimeConstant=0.001  UdotUserProvided=0
  Simulink-PS Converter4 : nesl_utility/Simulink-PS Converter  Commented=on  PhysicalDomain=network_engine_domain  SubClassName=ps_input  LeftPortType=input  RightPortType=output  PseudoPeriodic=off  Frequencies=[]  NoiseDistribution=none  NoiseParameters=[]  Unit=1  AffineConversion=off  FilteringAndDerivatives=filter  SimscapeFilterOrder=1  InputFilterTimeConstant=0.001  UdotUserProvided=0
  Simulink-PS Converter5 : nesl_utility/Simulink-PS Converter  Commented=on  PhysicalDomain=network_engine_domain  SubClassName=ps_input  LeftPortType=input  RightPortType=output  PseudoPeriodic=off  Frequencies=[]  NoiseDistribution=none  NoiseParameters=[]  Unit=1  AffineConversion=off  FilteringAndDerivatives=filter  SimscapeFilterOrder=1  InputFilterTimeConstant=0.001  UdotUserProvided=0
  Solver Configuration3 : nesl_utility/Solver Configuration  Commented=on  PhysicalDomain=network_engine_domain  SubClassName=solver  LeftPortType=input  RightPortType=generic  Tones=[]  Harmonics=[]  SimulateNoise=off  Profile=off  UseLocalSampling=off  EnableSwitchedLinearOptims=on  FrequencyDomain=off  UseCCode=off  RelTol=0.001  AbsTol=0.001  MinStep=1e-09  ToWorkspace=off  RevertToSquareIcSolve=off  NumHomotopyIterations=100  PhasorMode=off  PhasorModeNumHarmonics=1  ConsistencySolver=NEWTON_XTOL_AFTER_FTOL  IndexReductionMethod=DerivativeReplacement  DoDC=off  ResidualTolerance=1e-09  ConsistencyTolSource=GLOBAL  ConsistencyAbsTol=0.001  ConsistencyRelTol=0.001  ConsistencyTolFactor=0.001  UseLocalSolver=off  LocalSolverChoice=NE_BACKWARD_EULER_ADVANCER  ResolveIndetEquations=on  FunctionEvalNumThread=1  LocalSolverSampleTime=0.001  DoFixedCost=off  MaxNonlinIter=3  MaxModeIter=2  ComputeImpulses=off  ImpulseIterations=2  LinearAlgebra=auto  LinearAlgebraNumThread=0  EquationFormulation=NE_TIME_EF  DelaysMemoryBudget=1024  AutomaticFiltering=on  FilteringTimeConstant=0.001  PartitionStorageMethod=AS_NEEDED  PartitionMemoryBudget=1024  PartitionMethod=ROBUST  MultibodyUseLocalSolver=off  MultibodyLocalSolverChoice=ODE1  MultibodyLocalSolverSampleTime=0.001
  Step3 : Step  Commented=on  SampleTime=0
  Step4 : Step  Commented=on  SampleTime=0
  Step5 : Step  Commented=on  SampleTime=0
  Sum3 : Sum  Commented=on  Inputs=|+-
  Sum4 : Sum  Commented=on  Inputs=|+-
  Sum5 : Sum  Commented=on  Inputs=|+-
  World Frame3 : sm_lib/Frames and Transforms/World Frame  Commented=on
  wires:
  Sum5/1 -> Gain5/1
  Gain4/1 -> Simulink-PS Converter4/1
  PS-Simulink Converter4/1 -> Sum4/2
  Step5/1 -> Sum5/1
  Gain5/1 -> Simulink-PS Converter5/1
  Step4/1 -> Sum4/1
  Sum3/1 -> Gain3/1
  PS-Simulink Converter5/1 -> Sum5/2
  PS-Simulink Converter3/1 -> Sum3/2
  Step3/1 -> Sum3/1
  Sum4/1 -> Gain4/1
  Gain3/1 -> Simulink-PS Converter3/1
  connections:
  Revolute Joint11/LConn1 -- Rigid11/RConn1
  Simulink-PS Converter3/RConn1 -- Convertidor CD-CD/RConn1
  File Solid_12/RConn1 -- Rigid10/LConn1 -- Rigid9/RConn1
  Revolute Joint9/RConn3 -- Motor DC/LConn4
  Puente-H/LConn2 -- Convertidor CD-CD/LConn2
  Simulink-PS Converter4/RConn1 -- Convertidor CD-CD1/RConn1
  Revolute Joint11/RConn1 -- File Solid_11/RConn1
  Mechanism Configuration3/RConn1 -- Solver Configuration3/RConn1 -- Rigid9/LConn1 -- World Frame3/RConn1
  Motor DC2/LConn4 -- Revolute Joint11/RConn3
  Motor DC1/LConn4 -- Revolute Joint10/RConn3
  Puente-H2/RConn1 -- Motor DC2/LConn1
  Puente-H1/LConn2 -- Convertidor CD-CD1/LConn2
  PS-Simulink Converter4/LConn1 -- Revolute Joint10/RConn2
  Simulink-PS Converter5/RConn1 -- Convertidor CD-CD2/RConn1
  PS-Simulink Converter3/LConn1 -- Revolute Joint9/RConn2
  Puente-H2/LConn2 -- Convertidor CD-CD2/LConn2
  Motor DC2/LConn3 -- Revolute Joint11/LConn2
  Revolute Joint9/LConn1 -- Rigid3 2/RConn1
  File Solid_15/RConn1 -- Rigid11/LConn1 -- Revolute Joint10/RConn1
  Puente-H1/LConn1 -- Convertidor CD-CD1/LConn1
  Rigid12/LConn1 -- Revolute Joint9/RConn1 -- File Solid_14/RConn1
  Rigid3 2/LConn1 -- Rigid10/RConn1 -- File Solid_13/RConn1
  Puente-H/RConn1 -- Motor DC/LConn1
  Revolute Joint9/LConn2 -- Motor DC/LConn3
  Revolute Joint10/LConn1 -- Rigid12/RConn1
  Puente-H2/LConn1 -- Convertidor CD-CD2/LConn1
  Motor DC1/LConn3 -- Revolute Joint10/LConn2
  Puente-H1/RConn2 -- Motor DC1/LConn2
  PS-Simulink Converter5/LConn1 -- Revolute Joint11/RConn2
  Puente-H/RConn2 -- Motor DC/LConn2
  Puente-H/LConn1 -- Convertidor CD-CD/LConn1
  Puente-H1/RConn1 -- Motor DC1/LConn1
  Puente-H2/RConn2 -- Motor DC2/LConn2
